simulink subsystem "D2W4Test_sub"  (R2024b)
settings: Solver=VariableStepAuto  StartTime=0.0  StopTime=10.0  RelTol=1e-3
undefined symbols (not defined in the file): KePTR_k_TrcDvGain
settings Model: DefaultTestHarness=D2W4Test_sub_Harness1  Creator=StefanoCaserini  LastModifiedBy=StefanoLucaParravici
settings SolverCC: AlgebraicLoopSolver=TrustRegion
settings OptimizationCC: ReuseModelBlockBuffer=off
settings RTWCC: GPUComputeCapability=3.5  DLArmComputeVersion=19.05

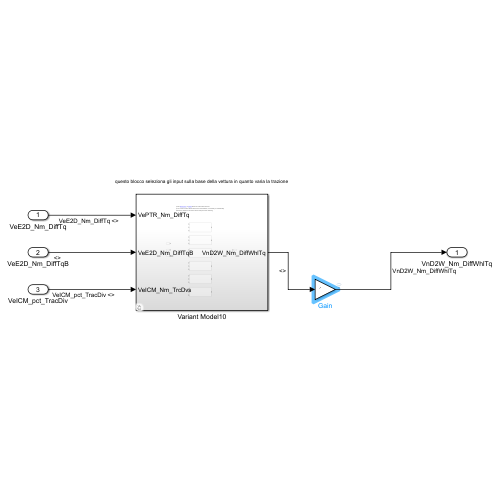
[thumbnail: Simulink's stored preview of the top-level diagram]
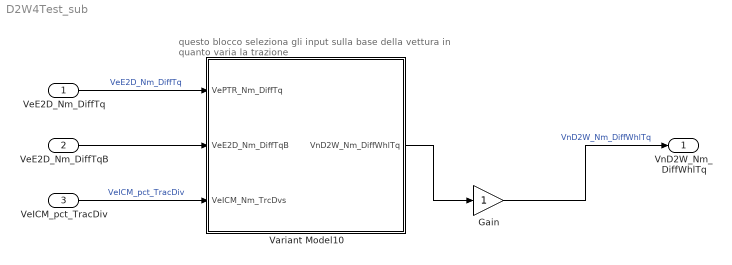
== system D2W4Test_sub ==
  note: questo blocco seleziona gli input sulla base della vettura in quanto varia la trazione
  VeE2D_Nm_DiffTq : Inport
  VeE2D_Nm_DiffTqB : Inport  Port=2
  VeICM_pct_TracDiv : Inport  Port=3
  Gain : Gain  OutDataTypeStr=Inherit: Same as input
  Variant Model10 : Subsystem  Variant=on  AllowZeroVariantControls=on
  VnD2W_Nm_DiffWhlTq : Outport  OutDataTypeStr=single  Unit=N*m  VectorParamsAs1DForOutWhenUnconnected=off
  wires:
  VeICM_pct_TracDiv/1 -> Variant Model10/3(VeICM_Nm_TrcDvs)  "VeICM_pct_TracDiv"
  VeE2D_Nm_DiffTq/1 -> Variant Model10/1(VePTR_Nm_DiffTq)  "VeE2D_Nm_DiffTq"
  Variant Model10/1(VnD2W_Nm_DiffWhlTq) -> Gain/1
  Gain/1 -> VnD2W_Nm_DiffWhlTq/1  "VnD2W_Nm_DiffWhlTq"
  VeE2D_Nm_DiffTqB/1 -> Variant Model10/2(VeE2D_Nm_DiffTqB)

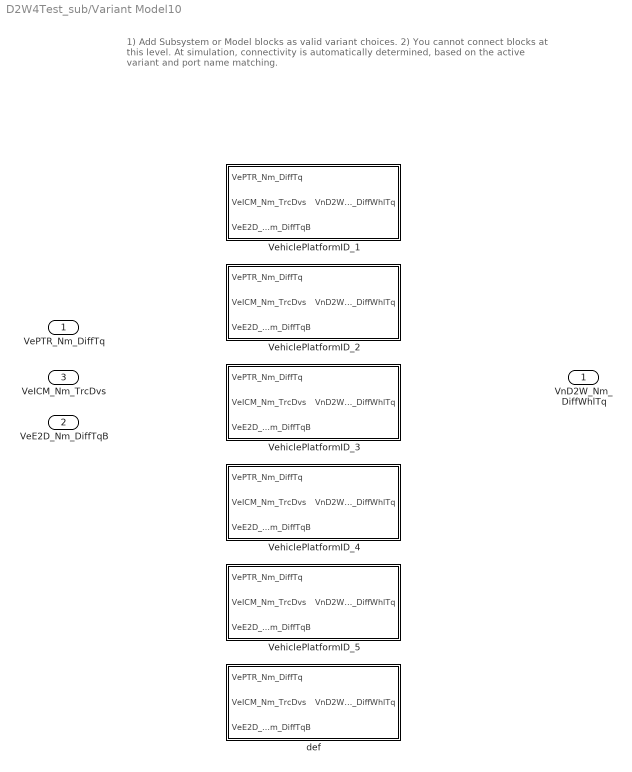
== system D2W4Test_sub/Variant Model10 ==
  note: 1) Add Subsystem or Model blocks as valid variant choices.
      | 2) You cannot connect blocks at this level. At simulation, connectivity is automatically
      | determined, based on the active variant and port name matching.
  VePTR_Nm_DiffTq : Inport
  VeE2D_Nm_DiffTqB : Inport  Port=2
  VeICM_Nm_TrcDvs : Inport  Port=3
  VehiclePlatformID_1 : Subsystem  TreatAsAtomicUnit=on  VariantControl=VehPtfm_ID == 1
  VehiclePlatformID_2 : Subsystem  TreatAsAtomicUnit=on  VariantControl=VehPtfm_ID == 2
  VehiclePlatformID_3 : Subsystem  TreatAsAtomicUnit=on  VariantControl=VehPtfm_ID == 3
  VehiclePlatformID_4 : Subsystem  TreatAsAtomicUnit=on  VariantControl=VehPtfm_ID == 4
  VehiclePlatformID_5 : Subsystem  TreatAsAtomicUnit=on  VariantControl=VehPtfm_ID == 5
  def : Subsystem  TreatAsAtomicUnit=on  VariantControl=(default)
  VnD2W_Nm_DiffWhlTq : Outport

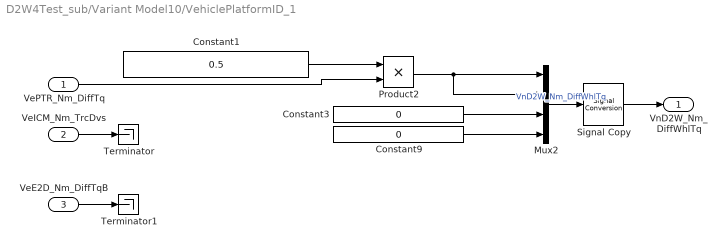
== system D2W4Test_sub/Variant Model10/VehiclePlatformID_1 ==
  VePTR_Nm_DiffTq : Inport
  VeICM_Nm_TrcDvs : Inport  Port=2
  VeE2D_Nm_DiffTqB : Inport  Port=3
  Constant1 : Constant  Value=0.5  OutDataTypeStr=Inherit: Inherit via back propagation  SampleTime=-1
  Constant3 : Constant  Value=0  OutDataTypeStr=Inherit: Inherit via back propagation  SampleTime=-1
  Constant9 : Constant  Value=0  OutDataTypeStr=Inherit: Inherit via back propagation  SampleTime=-1
  Mux2 : Mux
  Product2 : Product
  Signal Copy : SignalConversion  OverrideOpt=off
  Terminator : Terminator
  Terminator1 : Terminator
  VnD2W_Nm_DiffWhlTq : Outport
  wires:
  VeE2D_Nm_DiffTqB/1 -> Terminator1/1
  Product2/1 -> Mux2/2, Mux2/1
  Constant1/1 -> Product2/1
  Constant3/1 -> Mux2/3
  Mux2/1 -> Signal Copy/1  "VnD2W_Nm_DiffWhlTq"
  VePTR_Nm_DiffTq/1 -> Product2/2
  Constant9/1 -> Mux2/4
  VeICM_Nm_TrcDvs/1 -> Terminator/1
  Signal Copy/1 -> VnD2W_Nm_DiffWhlTq/1

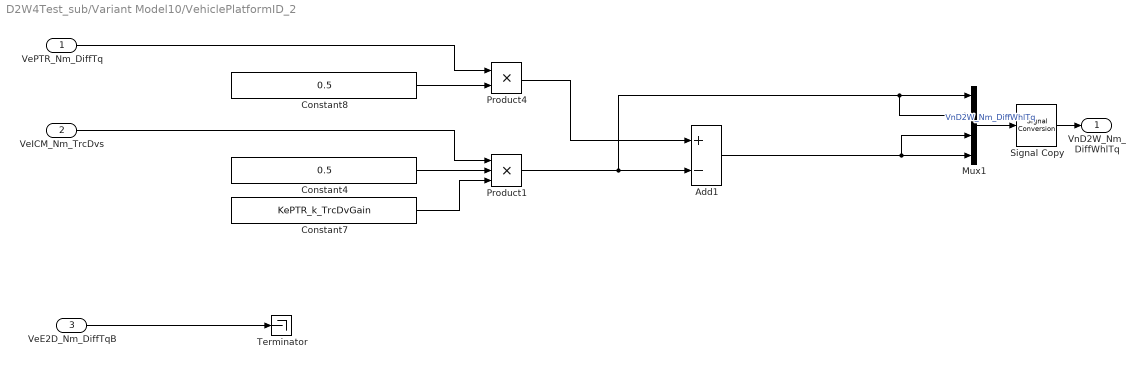
== system D2W4Test_sub/Variant Model10/VehiclePlatformID_2 ==
  VePTR_Nm_DiffTq : Inport
  VeICM_Nm_TrcDvs : Inport  Port=2
  VeE2D_Nm_DiffTqB : Inport  Port=3
  Add1 : Sum  Inputs=+-
  Constant4 : Constant  Value=0.5  OutDataTypeStr=Inherit: Inherit via back propagation  SampleTime=-1
  Constant7 : Constant  Value=KePTR_k_TrcDvGain  OutDataTypeStr=single  SampleTime=-1
  Constant8 : Constant  Value=0.5  OutDataTypeStr=Inherit: Inherit via back propagation  SampleTime=-1
  Mux1 : Mux
  Product1 : Product  Inputs=3
  Product4 : Product
  Signal Copy : SignalConversion  OverrideOpt=off
  Terminator : Terminator
  VnD2W_Nm_DiffWhlTq : Outport
  wires:
  VeE2D_Nm_DiffTqB/1 -> Terminator/1
  VePTR_Nm_DiffTq/1 -> Product4/1
  Add1/1 -> Mux1/3, Mux1/4
  Product4/1 -> Add1/1
  Product1/1 -> Mux1/1, Mux1/2, Add1/2
  Constant8/1 -> Product4/2
  Constant7/1 -> Product1/3
  VeICM_Nm_TrcDvs/1 -> Product1/1
  Constant4/1 -> Product1/2
  Mux1/1 -> Signal Copy/1  "VnD2W_Nm_DiffWhlTq"
  Signal Copy/1 -> VnD2W_Nm_DiffWhlTq/1

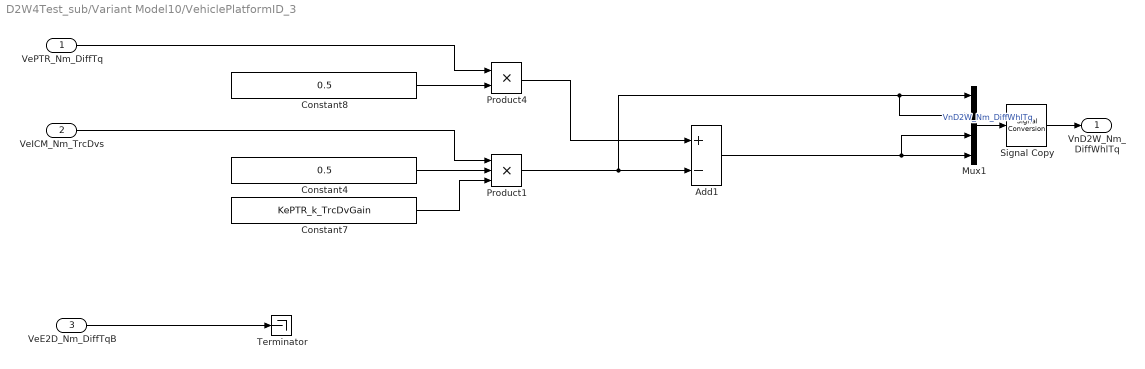
== system D2W4Test_sub/Variant Model10/VehiclePlatformID_3 ==
  VePTR_Nm_DiffTq : Inport
  VeICM_Nm_TrcDvs : Inport  Port=2
  VeE2D_Nm_DiffTqB : Inport  Port=3
  Add1 : Sum  Inputs=+-
  Constant4 : Constant  Value=0.5  OutDataTypeStr=Inherit: Inherit via back propagation  SampleTime=-1
  Constant7 : Constant  Value=KePTR_k_TrcDvGain  OutDataTypeStr=single  SampleTime=-1
  Constant8 : Constant  Value=0.5  OutDataTypeStr=Inherit: Inherit via back propagation  SampleTime=-1
  Mux1 : Mux
  Product1 : Product  Inputs=3
  Product4 : Product
  Signal Copy : SignalConversion  OverrideOpt=off
  Terminator : Terminator
  VnD2W_Nm_DiffWhlTq : Outport
  wires:
  Mux1/1 -> Signal Copy/1  "VnD2W_Nm_DiffWhlTq"
  Constant4/1 -> Product1/2
  VeICM_Nm_TrcDvs/1 -> Product1/1
  Constant7/1 -> Product1/3
  Constant8/1 -> Product4/2
  Product1/1 -> Add1/2, Mux1/2, Mux1/1
  Product4/1 -> Add1/1
  Add1/1 -> Mux1/4, Mux1/3
  VePTR_Nm_DiffTq/1 -> Product4/1
  VeE2D_Nm_DiffTqB/1 -> Terminator/1
  Signal Copy/1 -> VnD2W_Nm_DiffWhlTq/1

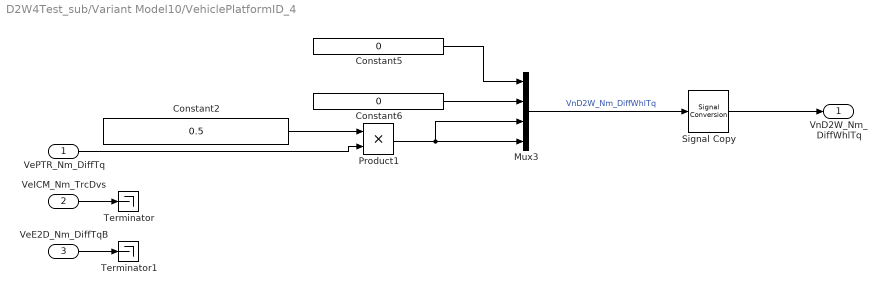
== system D2W4Test_sub/Variant Model10/VehiclePlatformID_4 ==
  VePTR_Nm_DiffTq : Inport
  VeICM_Nm_TrcDvs : Inport  Port=2
  VeE2D_Nm_DiffTqB : Inport  Port=3
  Constant2 : Constant  Value=0.5  OutDataTypeStr=Inherit: Inherit via back propagation  SampleTime=-1
  Constant5 : Constant  Value=0  OutDataTypeStr=Inherit: Inherit via back propagation  SampleTime=-1
  Constant6 : Constant  Value=0  OutDataTypeStr=Inherit: Inherit via back propagation  SampleTime=-1
  Mux3 : Mux
  Product1 : Product
  Signal Copy : SignalConversion  OverrideOpt=off
  Terminator : Terminator
  Terminator1 : Terminator
  VnD2W_Nm_DiffWhlTq : Outport
  wires:
  VeE2D_Nm_DiffTqB/1 -> Terminator1/1
  Product1/1 -> Mux3/3, Mux3/4
  VePTR_Nm_DiffTq/1 -> Product1/2
  Constant2/1 -> Product1/1
  Mux3/1 -> Signal Copy/1  "VnD2W_Nm_DiffWhlTq"
  Constant6/1 -> Mux3/2
  Constant5/1 -> Mux3/1
  VeICM_Nm_TrcDvs/1 -> Terminator/1
  Signal Copy/1 -> VnD2W_Nm_DiffWhlTq/1

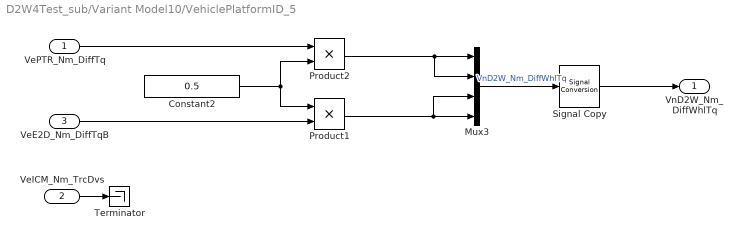
== system D2W4Test_sub/Variant Model10/VehiclePlatformID_5 ==
  VePTR_Nm_DiffTq : Inport
  VeICM_Nm_TrcDvs : Inport  Port=2
  VeE2D_Nm_DiffTqB : Inport  Port=3
  Constant2 : Constant  Value=0.5  OutDataTypeStr=Inherit: Inherit via back propagation  SampleTime=-1
  Mux3 : Mux
  Product1 : Product
  Product2 : Product
  Signal Copy : SignalConversion  OverrideOpt=off
  Terminator : Terminator
  VnD2W_Nm_DiffWhlTq : Outport
  wires:
  Product2/1 -> Mux3/1, Mux3/2
  VePTR_Nm_DiffTq/1 -> Product2/1
  VeICM_Nm_TrcDvs/1 -> Terminator/1
  Product1/1 -> Mux3/4, Mux3/3
  Mux3/1 -> Signal Copy/1  "VnD2W_Nm_DiffWhlTq"
  VeE2D_Nm_DiffTqB/1 -> Product1/2
  Constant2/1 -> Product1/1, Product2/2
  Signal Copy/1 -> VnD2W_Nm_DiffWhlTq/1

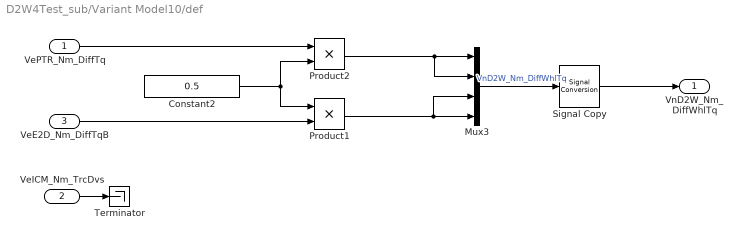
== system D2W4Test_sub/Variant Model10/def ==
  VePTR_Nm_DiffTq : Inport
  VeICM_Nm_TrcDvs : Inport  Port=2
  VeE2D_Nm_DiffTqB : Inport  Port=3
  Constant2 : Constant  Value=0.5  OutDataTypeStr=Inherit: Inherit via back propagation  SampleTime=-1
  Mux3 : Mux
  Product1 : Product
  Product2 : Product
  Signal Copy : SignalConversion  OverrideOpt=off
  Terminator : Terminator
  VnD2W_Nm_DiffWhlTq : Outport
  wires:
  Signal Copy/1 -> VnD2W_Nm_DiffWhlTq/1
  Constant2/1 -> Product2/2, Product1/1
  VeE2D_Nm_DiffTqB/1 -> Product1/2
  Mux3/1 -> Signal Copy/1  "VnD2W_Nm_DiffWhlTq"
  Product1/1 -> Mux3/3, Mux3/4
  VeICM_Nm_TrcDvs/1 -> Terminator/1
  VePTR_Nm_DiffTq/1 -> Product2/1
  Product2/1 -> Mux3/2, Mux3/1
